simulink model "Adaptive_Event_receive"  (R2023b)
settings: Solver=VariableStepAuto  StartTime=0.0  StopTime=10.0  RelTol=1e-3
libraries: autosarlibaprouting x1
settings Model: Creator=seame-workstation09  LastModifiedBy=seame-workstation09

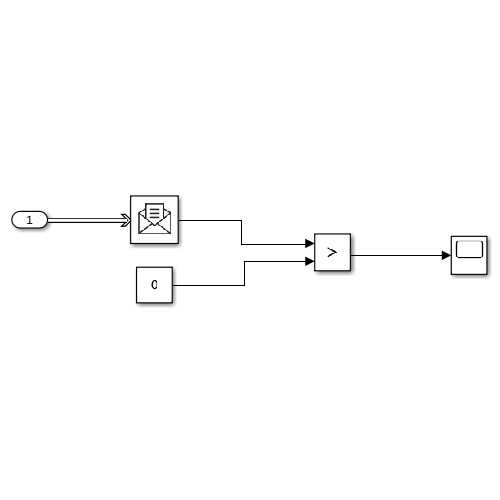
[thumbnail: Simulink's stored preview of the top-level diagram]
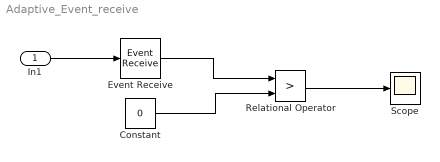
== system Adaptive_Event_receive ==
  In1 : Inport
  Constant : Constant  Value=0
  Event Receive : autosarlibaprouting/Event Receive
  Relational Operator : RelationalOperator  Operator=>  OutDataTypeStr=boolean  RndMeth=Simplest  InputSameDT=off
  Scope : Scope
  wires:
  In1/1 -> Event Receive/1
  Event Receive/1 -> Relational Operator/1
  Constant/1 -> Relational Operator/2
  Relational Operator/1 -> Scope/1
